simulink model "gm_uz_pmsm_model_9ph_21b_all_double_vnl"  (R2021b)
settings: Solver=FixedStepAuto  StartTime=0.0  StopTime=0.8  RelTol=1e-3
PreLoadFcn:
  | uz_pmsm_model_9ph_init_parameter
undefined symbols (not defined in the file or in its folder): a, b, c, friction_coefficient, inertia, k_i_d, k_i_q, k_p_d, k_p_q, Kpd, L_d, L_o1, L_o2, L_q, L_x1, L_x2, L_y1, L_y2, L_zero, polepair, psi_pm, R_1, static_friction_torque, Tnd, ts
libraries: hdlsllib x91, simulink x46, hdlmdlgenlib x17, dspsigops x7, slpidlib x2, spsAlphaBetaZerotodq0Lib x1, pid_lib x1, spsdq0toAlphaBetaZeroLib x1
(part 4 of 7)

== system gm_uz_pmsm_model_9ph_21b_all_double_vnl/uz_pmsm_model_9ph/abc_to_dq_vnl/Line-Line to Phase voltage ==
  u_abc1_pl : Inport
  Complex to Real-Imag : ComplexToRealImag
  Constant : Constant  Value=0  OutDataTypeStr=fixdt(1,25,12)  SampleTime=ts
  Constant1 : Constant  Value=1/sqrt(3)*exp(1i*-30/180*pi)  OutDataTypeStr=fixdt(1,18,16)  SampleTime=ts
  Demux3 : Demux  Outputs=3
  Mux4 : Mux  Inputs=3
  Product : Product  OutDataTypeStr=fixdt(1,25,12)
  Real-Imag to Complex : RealImagToComplex
  Terminator : Terminator
  abc   to   alpha_beta_0 : Subsystem
  alpha_beta_0   to   abc : Subsystem
  Out1 : Outport
  wires:
  Constant1/1 -> Product/2
  alpha_beta_0   to   abc/1("a, b, c") -> Out1/1
  abc   to   alpha_beta_0/1("alpha, beta, 0 ") -> Demux3/1
  Demux3/3 -> Terminator/1
  u_abc1_pl/1 -> abc   to   alpha_beta_0/1("a, b, c")
  Constant/1 -> Mux4/3
  Complex to Real-Imag/2 -> Mux4/2
  Demux3/1 -> Real-Imag to Complex/1
  Real-Imag to Complex/1 -> Product/1
  Product/1 -> Complex to Real-Imag/1
  Mux4/1 -> alpha_beta_0   to   abc/1("alpha, beta, 0  ")
  Complex to Real-Imag/1 -> Mux4/1
  Demux3/2 -> Real-Imag to Complex/2

== system gm_uz_pmsm_model_9ph_21b_all_double_vnl/uz_pmsm_model_9ph/abc_to_dq_vnl/Line-Line to Phase voltage1 ==
  u_abc2_pl : Inport
  Complex to Real-Imag : ComplexToRealImag
  Constant : Constant  Value=0  OutDataTypeStr=fixdt(1,25,12)  SampleTime=ts
  Constant1 : Constant  Value=1/sqrt(3)*exp(1i*-30/180*pi)  OutDataTypeStr=fixdt(1,18,16)  SampleTime=ts
  Demux3 : Demux  Outputs=3
  Mux4 : Mux  Inputs=3
  Product : Product  OutDataTypeStr=fixdt(1,25,12)
  Real-Imag to Complex : RealImagToComplex
  Terminator : Terminator
  abc   to   alpha_beta_0 : Subsystem
  alpha_beta_0   to   abc : Subsystem
  Out1 : Outport
  wires:
  Demux3/2 -> Real-Imag to Complex/2
  Complex to Real-Imag/1 -> Mux4/1
  Mux4/1 -> alpha_beta_0   to   abc/1("alpha, beta, 0  ")
  Product/1 -> Complex to Real-Imag/1
  Real-Imag to Complex/1 -> Product/1
  Demux3/1 -> Real-Imag to Complex/1
  Complex to Real-Imag/2 -> Mux4/2
  Constant/1 -> Mux4/3
  u_abc2_pl/1 -> abc   to   alpha_beta_0/1("a, b, c")
  Demux3/3 -> Terminator/1
  abc   to   alpha_beta_0/1("alpha, beta, 0 ") -> Demux3/1
  alpha_beta_0   to   abc/1("a, b, c") -> Out1/1
  Constant1/1 -> Product/2

== system gm_uz_pmsm_model_9ph_21b_all_double_vnl/uz_pmsm_model_9ph/abc_to_dq_vnl/Line-Line to Phase voltage2 ==
  u_abc3_pl : Inport
  Complex to Real-Imag : ComplexToRealImag
  Constant : Constant  Value=0  OutDataTypeStr=fixdt(1,25,12)  SampleTime=ts
  Constant1 : Constant  Value=1/sqrt(3)*exp(1i*-30/180*pi)  OutDataTypeStr=fixdt(1,18,16)  SampleTime=ts
  Demux3 : Demux  Outputs=3
  Mux4 : Mux  Inputs=3
  Product : Product  OutDataTypeStr=fixdt(1,25,12)
  Real-Imag to Complex : RealImagToComplex
  Terminator : Terminator
  abc   to   alpha_beta_0 : Subsystem
  alpha_beta_0   to   abc : Subsystem
  Out1 : Outport
  wires:
  Constant1/1 -> Product/2
  alpha_beta_0   to   abc/1("a, b, c") -> Out1/1
  abc   to   alpha_beta_0/1("alpha, beta, 0 ") -> Demux3/1
  Demux3/3 -> Terminator/1
  u_abc3_pl/1 -> abc   to   alpha_beta_0/1("a, b, c")
  Constant/1 -> Mux4/3
  Complex to Real-Imag/2 -> Mux4/2
  Demux3/1 -> Real-Imag to Complex/1
  Real-Imag to Complex/1 -> Product/1
  Product/1 -> Complex to Real-Imag/1
  Mux4/1 -> alpha_beta_0   to   abc/1("alpha, beta, 0  ")
  Complex to Real-Imag/1 -> Mux4/1
  Demux3/2 -> Real-Imag to Complex/2

== system gm_uz_pmsm_model_9ph_21b_all_double_vnl/uz_pmsm_model_9ph/abc_to_dq_vnl/Transformation ==
  in : Inport
  Add : Sum  OutDataTypeStr=fixdt(1,25,12)
  Add1 : Sum  Inputs=-+  OutDataTypeStr=fixdt(1,25,12)
  Constant1 : Constant  Value=c  OutDataTypeStr=fixdt(1,18,17)  SampleTime=ts
  Demux1 : Demux  Outputs=9
  Divide{,1..3} (4 alike) : Product  Inputs=**  OutDataTypeStr=fixdt(1,25,12)
  MatrixMultiply : Product  Multiplication=Matrix(*)  OutDataTypeStr=fixdt(1,25,12)
  Mux : Mux  Inputs=9
  out : Outport
  wires:
  in/1 -> MatrixMultiply/2
  MatrixMultiply/1 -> Demux1/1
  Constant1/1 -> MatrixMultiply/1
  Divide2/1 -> Add1/1
  Divide3/1 -> Add1/2
  [cos_theta_el] -> Divide3/1
  [sin_theta_el] -> Divide2/1
  [cos_theta_el] -> Divide/1  "cos_theta_hdl"
  [sin_theta_el] -> Divide1/1  "sin_theta_hdl"
  Divide1/1 -> Add/2
  Divide/1 -> Add/1
  Demux1/2 -> Divide3/2, Divide1/2  "u_beta"
  Demux1/1 -> Divide2/2, Divide/2  "u_alpha"
  Add/1 -> Mux/1
  Add1/1 -> Mux/2
  Mux/1 -> out/1  "trafo_out"
  Demux1/9 -> Mux/9
  Demux1/8 -> Mux/8
  Demux1/7 -> Mux/7
  Demux1/6 -> Mux/6
  Demux1/5 -> Mux/5
  Demux1/4 -> Mux/4
  Demux1/3 -> Mux/3

== system gm_uz_pmsm_model_9ph_21b_all_double_vnl/uz_pmsm_model_9ph/abc_to_dq_vnl/Transformation1 ==
  in : Inport
  Add : Sum  Inputs=+-  OutDataTypeStr=fixdt(1,25,12)
  Add1 : Sum  OutDataTypeStr=fixdt(1,25,12)
  Constant1 : Constant  Value=inv(c)  OutDataTypeStr=fixdt(1,18,16)  SampleTime=ts
  Data Type Conversion28 : DataTypeConversion  OutDataTypeStr=fixdt(1,25,12)  RndMeth=Nearest
  Demux1 : Demux  Outputs=9
  Divide{,1..3} (4 alike) : Product  Inputs=**  OutDataTypeStr=fixdt(1,25,12)
  MatrixMultiply : Product  Multiplication=Matrix(*)  OutDataTypeStr=fixdt(1,25,12)
  Mux : Mux  Inputs=9
  out : Outport
  wires:
  Data Type Conversion28/1 -> Demux1/1
  in/1 -> Data Type Conversion28/1
  MatrixMultiply/1 -> out/1
  Constant1/1 -> MatrixMultiply/1
  Mux/1 -> MatrixMultiply/2
  Add1/1 -> Mux/2
  [cos_theta_el] -> Divide3/1
  Divide2/1 -> Add1/1
  [sin_theta_el] -> Divide2/1
  Divide3/1 -> Add1/2
  Demux1/1 -> Divide/2, Divide2/2  "i_d"
  Divide1/1 -> Add/2
  [cos_theta_el] -> Divide/1
  Divide/1 -> Add/1
  Add/1 -> Mux/1
  Demux1/2 -> Divide1/2, Divide3/2  "i_q"
  [sin_theta_el] -> Divide1/1
  Demux1/7 -> Mux/7
  Demux1/9 -> Mux/9
  Demux1/5 -> Mux/5
  Demux1/3 -> Mux/3
  Demux1/4 -> Mux/4
  Demux1/6 -> Mux/6
  Demux1/8 -> Mux/8

== system gm_uz_pmsm_model_9ph_21b_all_double_vnl/uz_pmsm_model_9ph/dq_model_9ph/Wrapped State DTI ==
  note: https://de.mathworks.com/help/releases/R2021a/hdlcoder/ug/troubleshoot-generate-implementation-model-from-simscape-pmsm.html?searchHighlight=troubleshoot-generate-implementation-model-from-simscape-pmsm&s_tid=doc_srchtitle
  Angular Speed : Inport
  polepair : Inport  Port=2
  reset : Inport  Port=3
  Compare To Constant : simulink/Logic and Bit Operations/Compare To Constant  relop=>=  const=single(pi)  OutDataTypeStr=boolean
  Compare To Constant1 : simulink/Logic and Bit Operations/Compare To Constant  relop=<  const=single(-pi)  OutDataTypeStr=boolean
  Constant : Constant  Value=double(2*pi)  SampleTime=-1
  Delay1 : Delay  DelayLength=1  ExternalReset=Level
      settings: InputPortMap=u0,r5
  Gain : Gain  Gain=ts
  Product : Product
  Sum : Sum  Inputs=|++
  Sum1 : Sum  Inputs=|-+
  Sum2 : Sum  Inputs=|++
  Switch : Switch  Criteria=u2 > Threshold
  Switch1 : Switch  Criteria=u2 > Threshold
  Angular Position : Outport
  wires:
  polepair/1 -> Product/2
  Angular Speed/1 -> Product/1
  Product/1 -> Gain/1
  reset/1 -> Delay1/2
  Gain/1 -> Sum/2
  Sum1/1 -> Switch/1
  Sum/1 -> Switch/3, Sum1/2, Compare To Constant/1
  Compare To Constant/1 -> Switch/2
  Switch/1 -> Switch1/3, Compare To Constant1/1, Sum2/2
  Switch1/1 -> Delay1/1  "Angular Position"
  Sum2/1 -> Switch1/1
  Constant/1 -> Sum1/1, Sum2/1
  Delay1/1 -> Angular Position/1, Sum/1
  Compare To Constant1/1 -> Switch1/2

== system gm_uz_pmsm_model_9ph_21b_all_double_vnl/uz_pmsm_model_9ph/dq_model_9ph/mechanical_system ==
  note: This delay breaks the algebraic loop between mechanical and electrical system.
      | Introduces a delay of 500ns.
  note: load torque negative!!!
  reset : Inport
  M_Mi : Inport  Port=2
  reciprocal_J : Inport  Port=3
  load_torque : Inport  Port=4
  Delay : Delay  DelayLength=1
  Product11 : Product
  Sum1 : Sum  Inputs=|++
  integrator : Subsystem
  omega_mech : Outport
  wires:
  reset/1 -> integrator/2(reset)
  Product11/1 -> integrator/1(in)
  integrator/1(outt) -> omega_mech/1
  Delay/1 -> Sum1/1
  M_Mi/1 -> Delay/1
  load_torque/1 -> Sum1/2
  Sum1/1 -> Product11/2
  reciprocal_J/1 -> Product11/1

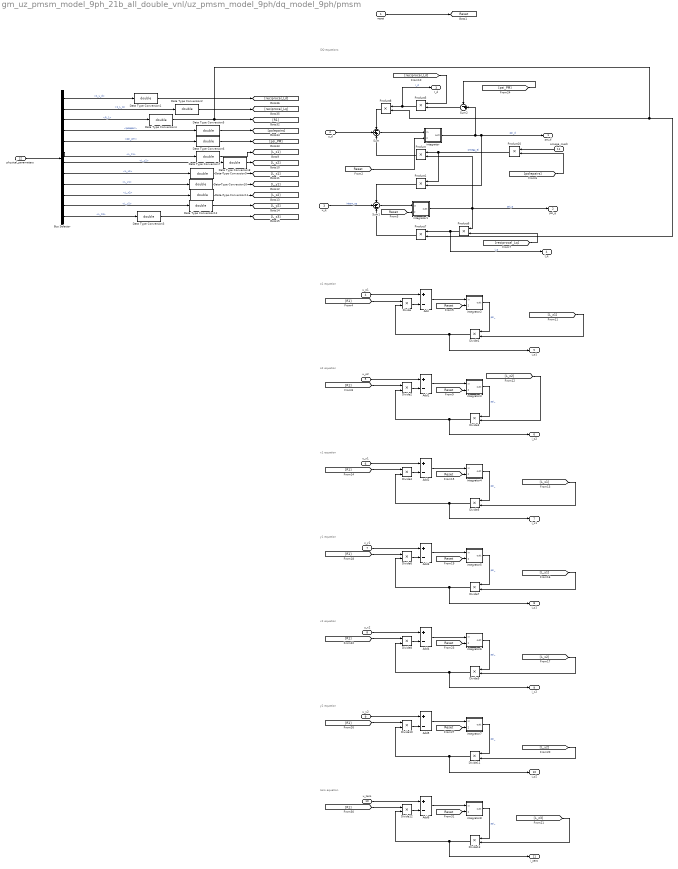
== system gm_uz_pmsm_model_9ph_21b_all_double_vnl/uz_pmsm_model_9ph/dq_model_9ph/pmsm ==
  note: zero equation
  note: y2 equation
  note: x2 equation
  note: y1 equation
  note: x1 equation
  note: o2 equation
  note: DQ equations
  note: o1 equation
  reset : Inport
  u_d : Inport  Port=2
  u_q : Inport  Port=3
  u_o1 : Inport  Port=4
  u_o2 : Inport  Port=5
  u_x1 : Inport  Port=6
  u_y1 : Inport  Port=7
  u_x2 : Inport  Port=8
  u_y2 : Inport  Port=9
  u_zero : Inport  Port=10
  omega_mech : Inport  Port=11
  physical_parameters : Inport  Port=12
  Add{,1..6} (7 alike) : Sum  Inputs=+-
  Bus Selector : BusSelector  OutputSignals=1_L_d,1_L_q,R_1,polepair,psi_pm,L_z1,L_z2,L_x1,L_y1,L_x2,L_y2,L_z3
  Data Type Conversion{1..12} (12 alike) : DataTypeConversion  OutDataTypeStr=double  RndMeth=Nearest
  Divide{,1..13} (14 alike) : Product  Inputs=**
  Product{,1,5..8,10} (7 alike) : Product
  Sum : Sum  Inputs=-++
  Sum1 : Sum  Inputs=-+-
  Sum2 : Sum  Inputs=-+|
  integrator : Subsystem
  integrator1 : Subsystem
  integrator2 : Subsystem
  integrator3 : Subsystem
  integrator4 : Subsystem
  integrator5 : Subsystem
  integrator6 : Subsystem
  integrator7 : Subsystem
  integrator8 : Subsystem
  psi_d : Outport
  psi_q : Outport  Port=2
  I_d : Outport  Port=3
  I_q : Outport  Port=4
  i_o1 : Outport  Port=5
  i_o2 : Outport  Port=6
  i_x1 : Outport  Port=7
  i_y1 : Outport  Port=8
  i_x2 : Outport  Port=9
  i_y2 : Outport  Port=10
  i_zero : Outport  Port=11
  tag scope: Reset=global
  wires:
  Data Type Conversion12/1 -> [L_y2]
  Data Type Conversion11/1 -> [L_x2]
  Data Type Conversion10/1 -> [L_y1]
  Data Type Conversion9/1 -> [L_x1]
  Data Type Conversion8/1 -> [L_z2]
  Data Type Conversion7/1 -> [L_z1]
  Data Type Conversion6/1 -> [psi_PM]
  Data Type Conversion5/1 -> [polepairs]
  Data Type Conversion4/1 -> Product8/2, Product7/2, [R1]
  Data Type Conversion2/1 -> [reciprocal_Lq]
  Bus Selector/12 -> Data Type Conversion3/1  "<L_z3>"
  Data Type Conversion3/1 -> [L_z3]
  Data Type Conversion1/1 -> [reciprocal_Ld]
  u_d/1 -> Sum/2
  Add6/1 -> integrator8/1(in)
  Add5/1 -> integrator7/1(in)
  Add4/1 -> integrator6/1(in)
  Add3/1 -> integrator5/1(in)
  Add2/1 -> integrator4/1(in)
  Add1/1 -> integrator3/1(in)
  Add/1 -> integrator2/1(in)
  Sum1/1 -> integrator1/1(in)
  Sum/1 -> integrator/1(in)
  [L_z3] -> Divide13/2
  [L_y2] -> Divide11/2
  [L_x2] -> Divide9/2
  [L_y1] -> Divide7/2
  [L_x1] -> Divide5/2
  [polepairs] -> Product10/2
  Bus Selector/9 -> Data Type Conversion10/1  "<L_y1>"
  physical_parameters/1 -> Bus Selector/1
  Bus Selector/10 -> Data Type Conversion11/1  "<L_x2>"
  Bus Selector/3 -> Data Type Conversion4/1  "<R_1>"
  Bus Selector/11 -> Data Type Conversion12/1  "<L_y2>"
  Bus Selector/7 -> Data Type Conversion8/1  "<L_z2>"
  Bus Selector/6 -> Data Type Conversion7/1  "<L_z1>"
  Bus Selector/5 -> Data Type Conversion6/1  "<psi_pm>"
  Bus Selector/2 -> Data Type Conversion2/1  "<1_L_q>"
  Bus Selector/8 -> Data Type Conversion9/1  "<L_x1>"
  Bus Selector/4 -> Data Type Conversion5/1  "<polepair>"
  Bus Selector/1 -> Data Type Conversion1/1  "<1_L_d>"
  integrator8/1(outt) -> Divide13/1  "psi_"
  [R1] -> Divide12/1
  Divide12/1 -> Add6/2
  Divide13/1 -> Divide12/2, i_zero/1
  u_zero/1 -> Add6/1
  [Reset] -> integrator8/2(reset)
  [Reset] -> integrator7/2(reset)
  u_y2/1 -> Add5/1
  Divide11/1 -> Divide10/2, i_y2/1
  Divide10/1 -> Add5/2
  [R1] -> Divide10/1
  integrator7/1(outt) -> Divide11/1  "psi_"
  integrator6/1(outt) -> Divide9/1  "psi_"
  [R1] -> Divide8/1
  Divide8/1 -> Add4/2
  Divide9/1 -> Divide8/2, i_x2/1
  u_x2/1 -> Add4/1
  [Reset] -> integrator6/2(reset)
  [Reset] -> integrator5/2(reset)
  u_y1/1 -> Add3/1
  Divide7/1 -> Divide6/2, i_y1/1
  Divide6/1 -> Add3/2
  [R1] -> Divide6/1
  integrator5/1(outt) -> Divide7/1  "psi_"
  integrator4/1(outt) -> Divide5/1  "psi_"
  [R1] -> Divide4/1
  Divide4/1 -> Add2/2
  Divide5/1 -> Divide4/2, i_x1/1
  u_x1/1 -> Add2/1
  [Reset] -> integrator4/2(reset)
  [Reset] -> integrator3/2(reset)
  [L_z2] -> Divide3/2
  u_o2/1 -> Add1/1
  Divide3/1 -> Divide2/2, i_o2/1
  Divide2/1 -> Add1/2
  [R1] -> Divide2/1
  integrator3/1(outt) -> Divide3/1  "psi_"
  integrator2/1(outt) -> Divide1/1  "psi_"
  [R1] -> Divide/1
  Divide/1 -> Add/2
  Divide1/1 -> Divide/2, i_o1/1
  u_o1/1 -> Add/1
  [L_z1] -> Divide1/2
  [Reset] -> integrator2/2(reset)
  [Reset] -> integrator1/2(reset)
  [Reset] -> integrator/2(reset)
  reset/1 -> [Reset]
  Product7/1 -> Sum1/3
  [reciprocal_Lq] -> Product6/2
  Product8/1 -> Sum/1
  Sum2/1 -> Product5/2
  integrator/1(outt) -> Product1/2, psi_d/1, Sum2/2  "psi_d"
  Product10/1 -> Product/1, Product1/1  "omega_el"
  Product6/1 -> Product7/1, I_q/1  "I_q"
  [psi_PM] -> Sum2/1
  Product1/1 -> Sum1/1
  integrator1/1(outt) -> Product6/1, Product/2, psi_q/1  "psi_q"
  [reciprocal_Ld] -> Product5/1
  Product5/1 -> Product8/1, I_d/1  "I_d"
  Product/1 -> Sum/3
  u_q/1 -> Sum1/2  "intern_uq"
  omega_mech/1 -> Product10/1

== system gm_uz_pmsm_model_9ph_21b_all_double_vnl/uz_pmsm_model_9ph/dq_model_9ph/torque_calculation ==
  I_d : Inport
  I_q : Inport  Port=2
  psi_d : Inport  Port=3
  psi_q : Inport  Port=4
  polepairs : Inport  Port=5
  Factor : Gain  Gain=9/2
  Product2 : Product
  Product3 : Product
  Product9 : Product
  Sum3 : Sum  Inputs=-|+
  M_Mi : Outport
  wires:
  Factor/1 -> Product9/1  "M_Mi"
  polepairs/1 -> Product9/2
  Product9/1 -> M_Mi/1  "M_Mi"
  I_q/1 -> Product3/2
  I_d/1 -> Product2/1
  psi_d/1 -> Product3/1
  psi_q/1 -> Product2/2
  Product2/1 -> Sum3/1
  Product3/1 -> Sum3/2
  Sum3/1 -> Factor/1

== system gm_uz_pmsm_model_9ph_21b_all_double_vnl/uz_pmsm_model_9ph/abc_to_dq/abc_to_dq/Divide ==
  in0 : Inport  OutDataTypeStr=fixdt(1, 17, 15)  SampleTime=1e-08
  in1 : Inport  Port=2  OutDataTypeStr=fixdt(1, 25, 12)  SampleTime=1e-08
  globalSchedule : EnablePort  OutDataTypeStr=boolean
  Divide : Product  Inputs=**  OutDataTypeStr=fixdt(1, 25, 12)  SampleTime=1e-08
  HwModeRegister : Delay  DelayLength=double(1)  InitialCondition=0
  HwModeRegister1 : Delay  DelayLength=double(1)  InitialCondition=0
  PipelineRegister : Delay  DelayLength=double(1)  InitialCondition=0
  out0 : Outport  OutDataTypeStr=fixdt(1, 25, 12)  SampleTime=1e-08  InitialOutput=0
  wires:
  HwModeRegister1/1 -> Divide/2
  HwModeRegister/1 -> Divide/1
  Divide/1 -> PipelineRegister/1
  in1/1 -> HwModeRegister1/1
  in0/1 -> HwModeRegister/1
  PipelineRegister/1 -> out0/1

== system gm_uz_pmsm_model_9ph_21b_all_double_vnl/uz_pmsm_model_9ph/abc_to_dq/abc_to_dq/Divide1 ==
  in0 : Inport  OutDataTypeStr=fixdt(1, 17, 15)  SampleTime=1e-08
  in1 : Inport  Port=2  OutDataTypeStr=fixdt(1, 25, 12)  SampleTime=1e-08
  globalSchedule : EnablePort  OutDataTypeStr=boolean
  Divide1 : Product  Inputs=**  OutDataTypeStr=fixdt(1, 25, 12)  SampleTime=1e-08
  HwModeRegister : Delay  DelayLength=double(1)  InitialCondition=0
  HwModeRegister1 : Delay  DelayLength=double(1)  InitialCondition=0
  PipelineRegister : Delay  DelayLength=double(1)  InitialCondition=0
  out0 : Outport  OutDataTypeStr=fixdt(1, 25, 12)  SampleTime=1e-08  InitialOutput=0
  wires:
  HwModeRegister1/1 -> Divide1/2
  HwModeRegister/1 -> Divide1/1
  Divide1/1 -> PipelineRegister/1
  in1/1 -> HwModeRegister1/1
  in0/1 -> HwModeRegister/1
  PipelineRegister/1 -> out0/1

== system gm_uz_pmsm_model_9ph_21b_all_double_vnl/uz_pmsm_model_9ph/abc_to_dq/abc_to_dq/Divide11 ==
  in0 : Inport  OutDataTypeStr=fixdt(1, 17, 15)  SampleTime=1e-08
  in1 : Inport  Port=2  OutDataTypeStr=fixdt(1, 25, 12)  SampleTime=1e-08
  globalSchedule : EnablePort  OutDataTypeStr=boolean
  Divide1 : Product  Inputs=**  OutDataTypeStr=fixdt(1, 25, 12)  SampleTime=1e-08
  HwModeRegister : Delay  DelayLength=double(1)  InitialCondition=0
  HwModeRegister1 : Delay  DelayLength=double(1)  InitialCondition=0
  PipelineRegister : Delay  DelayLength=double(1)  InitialCondition=0
  out0 : Outport  OutDataTypeStr=fixdt(1, 25, 12)  SampleTime=1e-08  InitialOutput=0
  wires:
  HwModeRegister1/1 -> Divide1/2
  HwModeRegister/1 -> Divide1/1
  Divide1/1 -> PipelineRegister/1
  in1/1 -> HwModeRegister1/1
  in0/1 -> HwModeRegister/1
  PipelineRegister/1 -> out0/1

== system gm_uz_pmsm_model_9ph_21b_all_double_vnl/uz_pmsm_model_9ph/abc_to_dq/abc_to_dq/Divide2 ==
  in0 : Inport  OutDataTypeStr=fixdt(1, 17, 15)  SampleTime=1e-08
  in1 : Inport  Port=2  OutDataTypeStr=fixdt(1, 25, 12)  SampleTime=1e-08
  globalSchedule : EnablePort  OutDataTypeStr=boolean
  Divide2 : Product  Inputs=**  OutDataTypeStr=fixdt(1, 25, 12)  SampleTime=1e-08
  HwModeRegister : Delay  DelayLength=double(1)  InitialCondition=0
  HwModeRegister1 : Delay  DelayLength=double(1)  InitialCondition=0
  PipelineRegister : Delay  DelayLength=double(1)  InitialCondition=0
  out0 : Outport  OutDataTypeStr=fixdt(1, 25, 12)  SampleTime=1e-08  InitialOutput=0
  wires:
  HwModeRegister1/1 -> Divide2/2
  HwModeRegister/1 -> Divide2/1
  Divide2/1 -> PipelineRegister/1
  in1/1 -> HwModeRegister1/1
  in0/1 -> HwModeRegister/1
  PipelineRegister/1 -> out0/1

== system gm_uz_pmsm_model_9ph_21b_all_double_vnl/uz_pmsm_model_9ph/abc_to_dq/abc_to_dq/Divide21 ==
  in0 : Inport  OutDataTypeStr=fixdt(1, 17, 15)  SampleTime=1e-08
  in1 : Inport  Port=2  OutDataTypeStr=fixdt(1, 25, 12)  SampleTime=1e-08
  globalSchedule : EnablePort  OutDataTypeStr=boolean
  Divide2 : Product  Inputs=**  OutDataTypeStr=fixdt(1, 25, 12)  SampleTime=1e-08
  HwModeRegister : Delay  DelayLength=double(1)  InitialCondition=0
  HwModeRegister1 : Delay  DelayLength=double(1)  InitialCondition=0
  PipelineRegister : Delay  DelayLength=double(1)  InitialCondition=0
  out0 : Outport  OutDataTypeStr=fixdt(1, 25, 12)  SampleTime=1e-08  InitialOutput=0
  wires:
  HwModeRegister1/1 -> Divide2/2
  HwModeRegister/1 -> Divide2/1
  Divide2/1 -> PipelineRegister/1
  in1/1 -> HwModeRegister1/1
  in0/1 -> HwModeRegister/1
  PipelineRegister/1 -> out0/1

== system gm_uz_pmsm_model_9ph_21b_all_double_vnl/uz_pmsm_model_9ph/abc_to_dq/abc_to_dq/Divide3 ==
  in0 : Inport  OutDataTypeStr=fixdt(1, 17, 15)  SampleTime=1e-08
  in1 : Inport  Port=2  OutDataTypeStr=fixdt(1, 25, 12)  SampleTime=1e-08
  globalSchedule : EnablePort  OutDataTypeStr=boolean
  Divide3 : Product  Inputs=**  OutDataTypeStr=fixdt(1, 25, 12)  SampleTime=1e-08
  HwModeRegister : Delay  DelayLength=double(1)  InitialCondition=0
  HwModeRegister1 : Delay  DelayLength=double(1)  InitialCondition=0
  PipelineRegister : Delay  DelayLength=double(1)  InitialCondition=0
  out0 : Outport  OutDataTypeStr=fixdt(1, 25, 12)  SampleTime=1e-08  InitialOutput=0
  wires:
  HwModeRegister1/1 -> Divide3/2
  HwModeRegister/1 -> Divide3/1
  Divide3/1 -> PipelineRegister/1
  in1/1 -> HwModeRegister1/1
  in0/1 -> HwModeRegister/1
  PipelineRegister/1 -> out0/1

== system gm_uz_pmsm_model_9ph_21b_all_double_vnl/uz_pmsm_model_9ph/abc_to_dq/abc_to_dq/Divide31 ==
  in0 : Inport  OutDataTypeStr=fixdt(1, 17, 15)  SampleTime=1e-08
  in1 : Inport  Port=2  OutDataTypeStr=fixdt(1, 25, 12)  SampleTime=1e-08
  globalSchedule : EnablePort  OutDataTypeStr=boolean
  Divide3 : Product  Inputs=**  OutDataTypeStr=fixdt(1, 25, 12)  SampleTime=1e-08
  HwModeRegister : Delay  DelayLength=double(1)  InitialCondition=0
  HwModeRegister1 : Delay  DelayLength=double(1)  InitialCondition=0
  PipelineRegister : Delay  DelayLength=double(1)  InitialCondition=0
  out0 : Outport  OutDataTypeStr=fixdt(1, 25, 12)  SampleTime=1e-08  InitialOutput=0
  wires:
  HwModeRegister1/1 -> Divide3/2
  HwModeRegister/1 -> Divide3/1
  Divide3/1 -> PipelineRegister/1
  in1/1 -> HwModeRegister1/1
  in0/1 -> HwModeRegister/1
  PipelineRegister/1 -> out0/1

== system gm_uz_pmsm_model_9ph_21b_all_double_vnl/uz_pmsm_model_9ph/abc_to_dq/abc_to_dq/Divide4 ==
  in0 : Inport  OutDataTypeStr=fixdt(1, 17, 15)  SampleTime=1e-08
  in1 : Inport  Port=2  OutDataTypeStr=fixdt(1, 25, 12)  SampleTime=1e-08
  globalSchedule : EnablePort  OutDataTypeStr=boolean
  Divide : Product  Inputs=**  OutDataTypeStr=fixdt(1, 25, 12)  SampleTime=1e-08
  HwModeRegister : Delay  DelayLength=double(1)  InitialCondition=0
  HwModeRegister1 : Delay  DelayLength=double(1)  InitialCondition=0
  PipelineRegister : Delay  DelayLength=double(1)  InitialCondition=0
  out0 : Outport  OutDataTypeStr=fixdt(1, 25, 12)  SampleTime=1e-08  InitialOutput=0
  wires:
  HwModeRegister1/1 -> Divide/2
  HwModeRegister/1 -> Divide/1
  Divide/1 -> PipelineRegister/1
  in1/1 -> HwModeRegister1/1
  in0/1 -> HwModeRegister/1
  PipelineRegister/1 -> out0/1

== system gm_uz_pmsm_model_9ph_21b_all_double_vnl/uz_pmsm_model_9ph/abc_to_dq/abc_to_dq/Gain ==
  in0 : Inport  OutDataTypeStr=fixdt(1, 18, 19)  SampleTime=1e-08
  in1 : Inport  Port=2  OutDataTypeStr=fixdt(1, 18, 14)  SampleTime=1e-08
  globalSchedule : EnablePort  OutDataTypeStr=boolean
  Gain : Product  Inputs=**  OutDataTypeStr=fixdt(1, 18, 16)  SampleTime=1e-08
  HwModeRegister : Delay  DelayLength=double(1)  InitialCondition=0
  HwModeRegister1 : Delay  DelayLength=double(1)  InitialCondition=0
  PipelineRegister : Delay  DelayLength=double(1)  InitialCondition=0
  out0 : Outport  OutDataTypeStr=fixdt(1, 18, 16)  SampleTime=1e-08  InitialOutput=0
  wires:
  HwModeRegister1/1 -> Gain/2
  HwModeRegister/1 -> Gain/1
  Gain/1 -> PipelineRegister/1
  in1/1 -> HwModeRegister1/1
  in0/1 -> HwModeRegister/1
  PipelineRegister/1 -> out0/1

== system gm_uz_pmsm_model_9ph_21b_all_double_vnl/uz_pmsm_model_9ph/abc_to_dq/abc_to_dq/Gain2 ==
  in0 : Inport  OutDataTypeStr=fixdt(1, 25, 12)  PortDimensions=[3]  SampleTime=1e-08
  in1 : Inport  Port=2  OutDataTypeStr=fixdt(1, 18, 16)  SampleTime=1e-08
  globalSchedule : EnablePort  OutDataTypeStr=boolean
  Gain2 : Product  Inputs=**  OutDataTypeStr=fixdt(1, 43, 28)  SampleTime=1e-08
  HwModeRegister : Delay  DelayLength=double(1)  InitialCondition=0
  HwModeRegister1 : Delay  DelayLength=double(1)  InitialCondition=0
  PipelineRegister : Delay  DelayLength=double(1)  InitialCondition=0
  out0 : Outport  OutDataTypeStr=fixdt(1, 43, 28)  PortDimensions=[3]  SampleTime=1e-08  InitialOutput=0
  wires:
  HwModeRegister1/1 -> Gain2/2
  HwModeRegister/1 -> Gain2/1
  Gain2/1 -> PipelineRegister/1
  in1/1 -> HwModeRegister1/1
  in0/1 -> HwModeRegister/1
  PipelineRegister/1 -> out0/1

== system gm_uz_pmsm_model_9ph_21b_all_double_vnl/uz_pmsm_model_9ph/abc_to_dq/abc_to_dq/Gain21 ==
  in0 : Inport  OutDataTypeStr=fixdt(1, 25, 12)  PortDimensions=[3]  SampleTime=1e-08
  in1 : Inport  Port=2  OutDataTypeStr=fixdt(1, 18, 16)  SampleTime=1e-08
  globalSchedule : EnablePort  OutDataTypeStr=boolean
  Gain2 : Product  Inputs=**  OutDataTypeStr=fixdt(1, 43, 28)  SampleTime=1e-08
  HwModeRegister : Delay  DelayLength=double(1)  InitialCondition=0
  HwModeRegister1 : Delay  DelayLength=double(1)  InitialCondition=0
  PipelineRegister : Delay  DelayLength=double(1)  InitialCondition=0
  out0 : Outport  OutDataTypeStr=fixdt(1, 43, 28)  PortDimensions=[3]  SampleTime=1e-08  InitialOutput=0
  wires:
  HwModeRegister1/1 -> Gain2/2
  HwModeRegister/1 -> Gain2/1
  Gain2/1 -> PipelineRegister/1
  in1/1 -> HwModeRegister1/1
  in0/1 -> HwModeRegister/1
  PipelineRegister/1 -> out0/1

== system gm_uz_pmsm_model_9ph_21b_all_double_vnl/uz_pmsm_model_9ph/abc_to_dq/abc_to_dq/Gain22 ==
  in0 : Inport  OutDataTypeStr=fixdt(1, 25, 12)  PortDimensions=[3]  SampleTime=1e-08
  in1 : Inport  Port=2  OutDataTypeStr=fixdt(1, 18, 16)  SampleTime=1e-08
  globalSchedule : EnablePort  OutDataTypeStr=boolean
  Gain2 : Product  Inputs=**  OutDataTypeStr=fixdt(1, 43, 28)  SampleTime=1e-08
  HwModeRegister : Delay  DelayLength=double(1)  InitialCondition=0
  HwModeRegister1 : Delay  DelayLength=double(1)  InitialCondition=0
  PipelineRegister : Delay  DelayLength=double(1)  InitialCondition=0
  out0 : Outport  OutDataTypeStr=fixdt(1, 43, 28)  PortDimensions=[3]  SampleTime=1e-08  InitialOutput=0
  wires:
  HwModeRegister1/1 -> Gain2/2
  HwModeRegister/1 -> Gain2/1
  Gain2/1 -> PipelineRegister/1
  in1/1 -> HwModeRegister1/1
  in0/1 -> HwModeRegister/1
  PipelineRegister/1 -> out0/1

== system gm_uz_pmsm_model_9ph_21b_all_double_vnl/uz_pmsm_model_9ph/abc_to_dq/abc_to_dq/MMul_dot_product ==
  in0 : Inport  OutDataTypeStr=fixdt(1, 18, 16)  PortDimensions=[9 1]  SampleTime=1e-08
  in1 : Inport  Port=2  OutDataTypeStr=fixdt(1, 25, 12)  PortDimensions=[9 1]  SampleTime=1e-08
  globalSchedule : EnablePort  OutDataTypeStr=boolean
  HwModeRegister : Delay  DelayLength=double(1)  InitialCondition=0
  HwModeRegister1 : Delay  DelayLength=double(1)  InitialCondition=0
  MMul_dot_product : Product  Inputs=**  OutDataTypeStr=fixdt(1, 43, 28)  SampleTime=1e-08
  PipelineRegister : Delay  DelayLength=double(1)  InitialCondition=0
  out0 : Outport  OutDataTypeStr=fixdt(1, 43, 28)  PortDimensions=[9 1]  SampleTime=1e-08  InitialOutput=0
  wires:
  HwModeRegister1/1 -> MMul_dot_product/2
  HwModeRegister/1 -> MMul_dot_product/1
  MMul_dot_product/1 -> PipelineRegister/1
  in1/1 -> HwModeRegister1/1
  in0/1 -> HwModeRegister/1
  PipelineRegister/1 -> out0/1

== system gm_uz_pmsm_model_9ph_21b_all_double_vnl/uz_pmsm_model_9ph/abc_to_dq/abc_to_dq/MMul_dot_product1 ==
  in0 : Inport  OutDataTypeStr=fixdt(1, 18, 16)  PortDimensions=[9 1]  SampleTime=1e-08
  in1 : Inport  Port=2  OutDataTypeStr=fixdt(1, 25, 12)  PortDimensions=[9 1]  SampleTime=1e-08
  globalSchedule : EnablePort  OutDataTypeStr=boolean
  HwModeRegister : Delay  DelayLength=double(1)  InitialCondition=0
  HwModeRegister1 : Delay  DelayLength=double(1)  InitialCondition=0
  MMul_dot_product : Product  Inputs=**  OutDataTypeStr=fixdt(1, 43, 28)  SampleTime=1e-08
  PipelineRegister : Delay  DelayLength=double(1)  InitialCondition=0
  out0 : Outport  OutDataTypeStr=fixdt(1, 43, 28)  PortDimensions=[9 1]  SampleTime=1e-08  InitialOutput=0
  wires:
  HwModeRegister1/1 -> MMul_dot_product/2
  HwModeRegister/1 -> MMul_dot_product/1
  MMul_dot_product/1 -> PipelineRegister/1
  in1/1 -> HwModeRegister1/1
  in0/1 -> HwModeRegister/1
  PipelineRegister/1 -> out0/1

== system gm_uz_pmsm_model_9ph_21b_all_double_vnl/uz_pmsm_model_9ph/abc_to_dq/abc_to_dq/MMul_dot_product2 ==
  in0 : Inport  OutDataTypeStr=fixdt(1, 18, 16)  PortDimensions=[9 1]  SampleTime=1e-08
  in1 : Inport  Port=2  OutDataTypeStr=fixdt(1, 25, 12)  PortDimensions=[9 1]  SampleTime=1e-08
  globalSchedule : EnablePort  OutDataTypeStr=boolean
  HwModeRegister : Delay  DelayLength=double(1)  InitialCondition=0
  HwModeRegister1 : Delay  DelayLength=double(1)  InitialCondition=0
  MMul_dot_product : Product  Inputs=**  OutDataTypeStr=fixdt(1, 43, 28)  SampleTime=1e-08
  PipelineRegister : Delay  DelayLength=double(1)  InitialCondition=0
  out0 : Outport  OutDataTypeStr=fixdt(1, 43, 28)  PortDimensions=[9 1]  SampleTime=1e-08  InitialOutput=0
  wires:
  HwModeRegister1/1 -> MMul_dot_product/2
  HwModeRegister/1 -> MMul_dot_product/1
  MMul_dot_product/1 -> PipelineRegister/1
  in1/1 -> HwModeRegister1/1
  in0/1 -> HwModeRegister/1
  PipelineRegister/1 -> out0/1

== system gm_uz_pmsm_model_9ph_21b_all_double_vnl/uz_pmsm_model_9ph/abc_to_dq/abc_to_dq/MMul_dot_product3 ==
  in0 : Inport  OutDataTypeStr=fixdt(1, 18, 16)  PortDimensions=[9 1]  SampleTime=1e-08
  in1 : Inport  Port=2  OutDataTypeStr=fixdt(1, 25, 12)  PortDimensions=[9 1]  SampleTime=1e-08
  globalSchedule : EnablePort  OutDataTypeStr=boolean
  HwModeRegister : Delay  DelayLength=double(1)  InitialCondition=0
  HwModeRegister1 : Delay  DelayLength=double(1)  InitialCondition=0
  MMul_dot_product : Product  Inputs=**  OutDataTypeStr=fixdt(1, 43, 28)  SampleTime=1e-08
  PipelineRegister : Delay  DelayLength=double(1)  InitialCondition=0
  out0 : Outport  OutDataTypeStr=fixdt(1, 43, 28)  PortDimensions=[9 1]  SampleTime=1e-08  InitialOutput=0
  wires:
  HwModeRegister1/1 -> MMul_dot_product/2
  HwModeRegister/1 -> MMul_dot_product/1
  MMul_dot_product/1 -> PipelineRegister/1
  in1/1 -> HwModeRegister1/1
  in0/1 -> HwModeRegister/1
  PipelineRegister/1 -> out0/1

== system gm_uz_pmsm_model_9ph_21b_all_double_vnl/uz_pmsm_model_9ph/abc_to_dq/abc_to_dq/MMul_dot_product4 ==
  in0 : Inport  OutDataTypeStr=fixdt(1, 18, 16)  PortDimensions=[9 1]  SampleTime=1e-08
  in1 : Inport  Port=2  OutDataTypeStr=fixdt(1, 25, 12)  PortDimensions=[9 1]  SampleTime=1e-08
  globalSchedule : EnablePort  OutDataTypeStr=boolean
  HwModeRegister : Delay  DelayLength=double(1)  InitialCondition=0
  HwModeRegister1 : Delay  DelayLength=double(1)  InitialCondition=0
  MMul_dot_product : Product  Inputs=**  OutDataTypeStr=fixdt(1, 43, 28)  SampleTime=1e-08
  PipelineRegister : Delay  DelayLength=double(1)  InitialCondition=0
  out0 : Outport  OutDataTypeStr=fixdt(1, 43, 28)  PortDimensions=[9 1]  SampleTime=1e-08  InitialOutput=0
  wires:
  HwModeRegister1/1 -> MMul_dot_product/2
  HwModeRegister/1 -> MMul_dot_product/1
  MMul_dot_product/1 -> PipelineRegister/1
  in1/1 -> HwModeRegister1/1
  in0/1 -> HwModeRegister/1
  PipelineRegister/1 -> out0/1

== system gm_uz_pmsm_model_9ph_21b_all_double_vnl/uz_pmsm_model_9ph/abc_to_dq/abc_to_dq/MMul_dot_product5 ==
  in0 : Inport  OutDataTypeStr=fixdt(1, 18, 16)  PortDimensions=[9 1]  SampleTime=1e-08
  in1 : Inport  Port=2  OutDataTypeStr=fixdt(1, 25, 12)  PortDimensions=[9 1]  SampleTime=1e-08
  globalSchedule : EnablePort  OutDataTypeStr=boolean
  HwModeRegister : Delay  DelayLength=double(1)  InitialCondition=0
  HwModeRegister1 : Delay  DelayLength=double(1)  InitialCondition=0
  MMul_dot_product : Product  Inputs=**  OutDataTypeStr=fixdt(1, 43, 28)  SampleTime=1e-08
  PipelineRegister : Delay  DelayLength=double(1)  InitialCondition=0
  out0 : Outport  OutDataTypeStr=fixdt(1, 43, 28)  PortDimensions=[9 1]  SampleTime=1e-08  InitialOutput=0
  wires:
  HwModeRegister1/1 -> MMul_dot_product/2
  HwModeRegister/1 -> MMul_dot_product/1
  MMul_dot_product/1 -> PipelineRegister/1
  in1/1 -> HwModeRegister1/1
  in0/1 -> HwModeRegister/1
  PipelineRegister/1 -> out0/1

== system gm_uz_pmsm_model_9ph_21b_all_double_vnl/uz_pmsm_model_9ph/abc_to_dq/abc_to_dq/Product ==
  in0 : Inport  OutDataTypeStr=fixdt(1, 25, 12)  SampleTime=1e-08
  in1 : Inport  Port=2  OutDataTypeStr=fixdt(1, 18, 16)  SampleTime=1e-08
  globalSchedule : EnablePort  OutDataTypeStr=boolean
  HwModeRegister : Delay  DelayLength=double(1)  InitialCondition=0
  HwModeRegister1 : Delay  DelayLength=double(1)  InitialCondition=0
  PipelineRegister : Delay  DelayLength=double(1)  InitialCondition=0
  Product : Product  Inputs=**  OutDataTypeStr=fixdt(1, 25, 12)  SampleTime=1e-08
  out0 : Outport  OutDataTypeStr=fixdt(1, 25, 12)  SampleTime=1e-08  InitialOutput=0
  wires:
  HwModeRegister1/1 -> Product/2
  HwModeRegister/1 -> Product/1
  Product/1 -> PipelineRegister/1
  in1/1 -> HwModeRegister1/1
  in0/1 -> HwModeRegister/1
  PipelineRegister/1 -> out0/1

== system gm_uz_pmsm_model_9ph_21b_all_double_vnl/uz_pmsm_model_9ph/abc_to_dq/abc_to_dq/Product1 ==
  in0 : Inport  OutDataTypeStr=fixdt(1, 25, 12)  SampleTime=1e-08
  in1 : Inport  Port=2  OutDataTypeStr=fixdt(1, 18, 16)  SampleTime=1e-08
  globalSchedule : EnablePort  OutDataTypeStr=boolean
  HwModeRegister : Delay  DelayLength=double(1)  InitialCondition=0
  HwModeRegister1 : Delay  DelayLength=double(1)  InitialCondition=0
  PipelineRegister : Delay  DelayLength=double(1)  InitialCondition=0
  Product : Product  Inputs=**  OutDataTypeStr=fixdt(1, 25, 12)  SampleTime=1e-08
  out0 : Outport  OutDataTypeStr=fixdt(1, 25, 12)  SampleTime=1e-08  InitialOutput=0
  wires:
  HwModeRegister1/1 -> Product/2
  HwModeRegister/1 -> Product/1
  Product/1 -> PipelineRegister/1
  in1/1 -> HwModeRegister1/1
  in0/1 -> HwModeRegister/1
  PipelineRegister/1 -> out0/1

== system gm_uz_pmsm_model_9ph_21b_all_double_vnl/uz_pmsm_model_9ph/abc_to_dq/abc_to_dq/Product10 ==
  in0 : Inport  OutDataTypeStr=fixdt(1, 25, 12)  SampleTime=1e-08
  in1 : Inport  Port=2  OutDataTypeStr=fixdt(1, 18, 16)  SampleTime=1e-08
  globalSchedule : EnablePort  OutDataTypeStr=boolean
  HwModeRegister : Delay  DelayLength=double(1)  InitialCondition=0
  HwModeRegister1 : Delay  DelayLength=double(1)  InitialCondition=0
  PipelineRegister : Delay  DelayLength=double(1)  InitialCondition=0
  Product : Product  Inputs=**  OutDataTypeStr=fixdt(1, 25, 12)  SampleTime=1e-08
  out0 : Outport  OutDataTypeStr=fixdt(1, 25, 12)  SampleTime=1e-08  InitialOutput=0
  wires:
  HwModeRegister1/1 -> Product/2
  HwModeRegister/1 -> Product/1
  Product/1 -> PipelineRegister/1
  in1/1 -> HwModeRegister1/1
  in0/1 -> HwModeRegister/1
  PipelineRegister/1 -> out0/1

== system gm_uz_pmsm_model_9ph_21b_all_double_vnl/uz_pmsm_model_9ph/abc_to_dq/abc_to_dq/Product11 ==
  in0 : Inport  OutDataTypeStr=fixdt(1, 25, 12)  SampleTime=1e-08
  in1 : Inport  Port=2  OutDataTypeStr=fixdt(1, 18, 16)  SampleTime=1e-08
  globalSchedule : EnablePort  OutDataTypeStr=boolean
  HwModeRegister : Delay  DelayLength=double(1)  InitialCondition=0
  HwModeRegister1 : Delay  DelayLength=double(1)  InitialCondition=0
  PipelineRegister : Delay  DelayLength=double(1)  InitialCondition=0
  Product : Product  Inputs=**  OutDataTypeStr=fixdt(1, 25, 12)  SampleTime=1e-08
  out0 : Outport  OutDataTypeStr=fixdt(1, 25, 12)  SampleTime=1e-08  InitialOutput=0
  wires:
  HwModeRegister1/1 -> Product/2
  HwModeRegister/1 -> Product/1
  Product/1 -> PipelineRegister/1
  in1/1 -> HwModeRegister1/1
  in0/1 -> HwModeRegister/1
  PipelineRegister/1 -> out0/1

== system gm_uz_pmsm_model_9ph_21b_all_double_vnl/uz_pmsm_model_9ph/abc_to_dq/abc_to_dq/Product2 ==
  in0 : Inport  OutDataTypeStr=fixdt(1, 25, 12)  SampleTime=1e-08
  in1 : Inport  Port=2  OutDataTypeStr=fixdt(1, 18, 16)  SampleTime=1e-08
  globalSchedule : EnablePort  OutDataTypeStr=boolean
  HwModeRegister : Delay  DelayLength=double(1)  InitialCondition=0
  HwModeRegister1 : Delay  DelayLength=double(1)  InitialCondition=0
  PipelineRegister : Delay  DelayLength=double(1)  InitialCondition=0
  Product : Product  Inputs=**  OutDataTypeStr=fixdt(1, 25, 12)  SampleTime=1e-08
  out0 : Outport  OutDataTypeStr=fixdt(1, 25, 12)  SampleTime=1e-08  InitialOutput=0
  wires:
  HwModeRegister1/1 -> Product/2
  HwModeRegister/1 -> Product/1
  Product/1 -> PipelineRegister/1
  in1/1 -> HwModeRegister1/1
  in0/1 -> HwModeRegister/1
  PipelineRegister/1 -> out0/1

== system gm_uz_pmsm_model_9ph_21b_all_double_vnl/uz_pmsm_model_9ph/abc_to_dq/abc_to_dq/Product3 ==
  in0 : Inport  OutDataTypeStr=fixdt(1, 25, 12)  SampleTime=1e-08
  in1 : Inport  Port=2  OutDataTypeStr=fixdt(1, 18, 16)  SampleTime=1e-08
  globalSchedule : EnablePort  OutDataTypeStr=boolean
  HwModeRegister : Delay  DelayLength=double(1)  InitialCondition=0
  HwModeRegister1 : Delay  DelayLength=double(1)  InitialCondition=0
  PipelineRegister : Delay  DelayLength=double(1)  InitialCondition=0
  Product : Product  Inputs=**  OutDataTypeStr=fixdt(1, 25, 12)  SampleTime=1e-08
  out0 : Outport  OutDataTypeStr=fixdt(1, 25, 12)  SampleTime=1e-08  InitialOutput=0
  wires:
  HwModeRegister1/1 -> Product/2
  HwModeRegister/1 -> Product/1
  Product/1 -> PipelineRegister/1
  in1/1 -> HwModeRegister1/1
  in0/1 -> HwModeRegister/1
  PipelineRegister/1 -> out0/1

== system gm_uz_pmsm_model_9ph_21b_all_double_vnl/uz_pmsm_model_9ph/abc_to_dq/abc_to_dq/Product4 ==
  in0 : Inport  OutDataTypeStr=fixdt(1, 25, 12)  SampleTime=1e-08
  in1 : Inport  Port=2  OutDataTypeStr=fixdt(1, 18, 16)  SampleTime=1e-08
  globalSchedule : EnablePort  OutDataTypeStr=boolean
  HwModeRegister : Delay  DelayLength=double(1)  InitialCondition=0
  HwModeRegister1 : Delay  DelayLength=double(1)  InitialCondition=0
  PipelineRegister : Delay  DelayLength=double(1)  InitialCondition=0
  Product : Product  Inputs=**  OutDataTypeStr=fixdt(1, 25, 12)  SampleTime=1e-08
  out0 : Outport  OutDataTypeStr=fixdt(1, 25, 12)  SampleTime=1e-08  InitialOutput=0
  wires:
  HwModeRegister1/1 -> Product/2
  HwModeRegister/1 -> Product/1
  Product/1 -> PipelineRegister/1
  in1/1 -> HwModeRegister1/1
  in0/1 -> HwModeRegister/1
  PipelineRegister/1 -> out0/1

== system gm_uz_pmsm_model_9ph_21b_all_double_vnl/uz_pmsm_model_9ph/abc_to_dq/abc_to_dq/Product5 ==
  in0 : Inport  OutDataTypeStr=fixdt(1, 25, 12)  SampleTime=1e-08
  in1 : Inport  Port=2  OutDataTypeStr=fixdt(1, 18, 16)  SampleTime=1e-08
  globalSchedule : EnablePort  OutDataTypeStr=boolean
  HwModeRegister : Delay  DelayLength=double(1)  InitialCondition=0
  HwModeRegister1 : Delay  DelayLength=double(1)  InitialCondition=0
  PipelineRegister : Delay  DelayLength=double(1)  InitialCondition=0
  Product : Product  Inputs=**  OutDataTypeStr=fixdt(1, 25, 12)  SampleTime=1e-08
  out0 : Outport  OutDataTypeStr=fixdt(1, 25, 12)  SampleTime=1e-08  InitialOutput=0
  wires:
  HwModeRegister1/1 -> Product/2
  HwModeRegister/1 -> Product/1
  Product/1 -> PipelineRegister/1
  in1/1 -> HwModeRegister1/1
  in0/1 -> HwModeRegister/1
  PipelineRegister/1 -> out0/1

== system gm_uz_pmsm_model_9ph_21b_all_double_vnl/uz_pmsm_model_9ph/abc_to_dq/abc_to_dq/Product6 ==
  in0 : Inport  OutDataTypeStr=fixdt(1, 25, 12)  SampleTime=1e-08
  in1 : Inport  Port=2  OutDataTypeStr=fixdt(1, 18, 16)  SampleTime=1e-08
  globalSchedule : EnablePort  OutDataTypeStr=boolean
  HwModeRegister : Delay  DelayLength=double(1)  InitialCondition=0
  HwModeRegister1 : Delay  DelayLength=double(1)  InitialCondition=0
  PipelineRegister : Delay  DelayLength=double(1)  InitialCondition=0
  Product : Product  Inputs=**  OutDataTypeStr=fixdt(1, 25, 12)  SampleTime=1e-08
  out0 : Outport  OutDataTypeStr=fixdt(1, 25, 12)  SampleTime=1e-08  InitialOutput=0
  wires:
  HwModeRegister1/1 -> Product/2
  HwModeRegister/1 -> Product/1
  Product/1 -> PipelineRegister/1
  in1/1 -> HwModeRegister1/1
  in0/1 -> HwModeRegister/1
  PipelineRegister/1 -> out0/1

== system gm_uz_pmsm_model_9ph_21b_all_double_vnl/uz_pmsm_model_9ph/abc_to_dq/abc_to_dq/Product7 ==
  in0 : Inport  OutDataTypeStr=fixdt(1, 25, 12)  SampleTime=1e-08
  in1 : Inport  Port=2  OutDataTypeStr=fixdt(1, 18, 16)  SampleTime=1e-08
  globalSchedule : EnablePort  OutDataTypeStr=boolean
  HwModeRegister : Delay  DelayLength=double(1)  InitialCondition=0
  HwModeRegister1 : Delay  DelayLength=double(1)  InitialCondition=0
  PipelineRegister : Delay  DelayLength=double(1)  InitialCondition=0
  Product : Product  Inputs=**  OutDataTypeStr=fixdt(1, 25, 12)  SampleTime=1e-08
  out0 : Outport  OutDataTypeStr=fixdt(1, 25, 12)  SampleTime=1e-08  InitialOutput=0
  wires:
  HwModeRegister1/1 -> Product/2
  HwModeRegister/1 -> Product/1
  Product/1 -> PipelineRegister/1
  in1/1 -> HwModeRegister1/1
  in0/1 -> HwModeRegister/1
  PipelineRegister/1 -> out0/1

== system gm_uz_pmsm_model_9ph_21b_all_double_vnl/uz_pmsm_model_9ph/abc_to_dq/abc_to_dq/Product8 ==
  in0 : Inport  OutDataTypeStr=fixdt(1, 25, 12)  SampleTime=1e-08
  in1 : Inport  Port=2  OutDataTypeStr=fixdt(1, 18, 16)  SampleTime=1e-08
  globalSchedule : EnablePort  OutDataTypeStr=boolean
  HwModeRegister : Delay  DelayLength=double(1)  InitialCondition=0
  HwModeRegister1 : Delay  DelayLength=double(1)  InitialCondition=0
  PipelineRegister : Delay  DelayLength=double(1)  InitialCondition=0
  Product : Product  Inputs=**  OutDataTypeStr=fixdt(1, 25, 12)  SampleTime=1e-08
  out0 : Outport  OutDataTypeStr=fixdt(1, 25, 12)  SampleTime=1e-08  InitialOutput=0
  wires:
  HwModeRegister1/1 -> Product/2
  HwModeRegister/1 -> Product/1
  Product/1 -> PipelineRegister/1
  in1/1 -> HwModeRegister1/1
  in0/1 -> HwModeRegister/1
  PipelineRegister/1 -> out0/1

== system gm_uz_pmsm_model_9ph_21b_all_double_vnl/uz_pmsm_model_9ph/abc_to_dq/abc_to_dq/Product9 ==
  in0 : Inport  OutDataTypeStr=fixdt(1, 25, 12)  SampleTime=1e-08
  in1 : Inport  Port=2  OutDataTypeStr=fixdt(1, 18, 16)  SampleTime=1e-08
  globalSchedule : EnablePort  OutDataTypeStr=boolean
  HwModeRegister : Delay  DelayLength=double(1)  InitialCondition=0
  HwModeRegister1 : Delay  DelayLength=double(1)  InitialCondition=0
  PipelineRegister : Delay  DelayLength=double(1)  InitialCondition=0
  Product : Product  Inputs=**  OutDataTypeStr=fixdt(1, 25, 12)  SampleTime=1e-08
  out0 : Outport  OutDataTypeStr=fixdt(1, 25, 12)  SampleTime=1e-08  InitialOutput=0
  wires:
  HwModeRegister1/1 -> Product/2
  HwModeRegister/1 -> Product/1
  Product/1 -> PipelineRegister/1
  in1/1 -> HwModeRegister1/1
  in0/1 -> HwModeRegister/1
  PipelineRegister/1 -> out0/1
